simulink model "EdgeDetect"  (R2018b)
settings: Solver=VariableStepAuto  StartTime=0.0  StopTime=(64*3)*320e-9  RelTol=1e-3
libraries: xbsIndex_r4 x16, simulink_extras x2
settings Model: Creator=marsiau  LastModifiedBy=marsiau

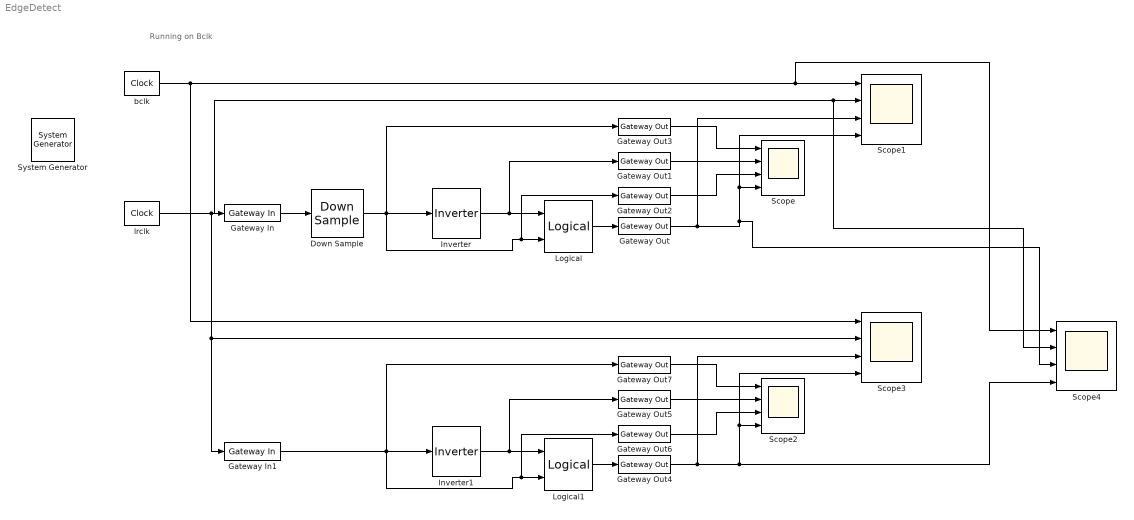
== system EdgeDetect ==
  note: Running on Bclk
  " System Generator" : xbsIndex_r4/ System Generator  Tag=genX  xilinxfamily=zynq  part=xc7z020  speed=-1  package=clg400  synthesis_tool=Vivado  clock_wrapper=Clock Enables  directory=./netlist  proj_type=Vivado  Synth_file=Vivado Synthesis Defaults  Impl_file=Vivado Implementation Defaults  testbench=off  simulink_period=320e-9  sysclk_period=320  dcm_input_clock_period=10  incr_netlist=off  trim_vbits=Everywhere in SubSystem  dbl_ovrd=According to Block Masks  core_generation=According to Block Masks  run_coregen=off  deprecated_control=off  eval_field=0  block_type=sysgen
  Down Sample : xbsIndex_r4/Down Sample  sample_ratio=32  sample_phase="Last Value of Frame  (most efficient)"  en=off  rst=off  latency=1  dbl_ovrd=off  block_type=dsamp
  Gateway In : xbsIndex_r4/Gateway In  gui_display_data_type=Boolean  arith_type=Boolean  n_bits=16  bin_pt=14  preci_type=Single  exp_width=8  frac_width=24  rows=1  columns=1  quantization="Round  (unbiased: +/- Inf)"  overflow=Saturate  period=320e-9  UseAsADC=off  ADCChannel='1'  interface=None  automatic_assignment=on  address_offset=hex2dec('00')  intf_name=''  intf_description=''  default_value=0  timing_constraint=None  locs_specified=off  LOCs={}  io_standard={}  inherit_from_input=off  hdl_port=on  dbl_ovrd=off  block_type=gatewayin
  Gateway In1 : xbsIndex_r4/Gateway In  gui_display_data_type=Boolean  arith_type=Boolean  n_bits=16  bin_pt=14  preci_type=Single  exp_width=8  frac_width=24  rows=1  columns=1  quantization="Round  (unbiased: +/- Inf)"  overflow=Saturate  period=320e-9  UseAsADC=off  ADCChannel='1'  interface=None  automatic_assignment=on  address_offset=hex2dec('00')  intf_name=''  intf_description=''  default_value=0  timing_constraint=None  locs_specified=off  LOCs={}  io_standard={}  inherit_from_input=off  hdl_port=on  dbl_ovrd=off  block_type=gatewayin
  Gateway Out{,1..7} (8 alike) : xbsIndex_r4/Gateway Out  inherit_from_input=off  hdl_port=on  rows=1  columns=1  UseAsDAC=off  DACChannel='1'  interface=None  automatic_assignment=on  address_offset=hex2dec('00')  intf_name=''  intf_description=''  timing_constraint=None  locs_specified=off  LOCs={}  io_standard={}  block_type=gatewayout
  Inverter : xbsIndex_r4/Inverter  en=off  latency=1  dbl_ovrd=off  block_type=inv
  Inverter1 : xbsIndex_r4/Inverter  en=off  latency=1  dbl_ovrd=off  block_type=inv
  Logical : xbsIndex_r4/Logical  logical_function=AND  inputs=2  en=off  latency=1  precision=Full  arith_type=Unsigned  n_bits=16  bin_pt=0  align_bp=on  dbl_ovrd=off  block_type=logical
  Logical1 : xbsIndex_r4/Logical  logical_function=AND  inputs=2  en=off  latency=1  precision=Full  arith_type=Unsigned  n_bits=16  bin_pt=0  align_bp=on  dbl_ovrd=off  block_type=logical
  Scope{,1..4} (5 alike) : Scope  NumInputPorts=4
  bclk : simulink_extras/Flip Flops/Clock  period=320e-9
  lrclk : simulink_extras/Flip Flops/Clock  period=20.48e-6
  wires:
  Logical/1 -> Gateway Out/1
  Inverter/1 -> Gateway Out1/1, Logical/1
  Gateway In/1 -> Down Sample/1
  Gateway Out3/1 -> Scope/1
  Gateway Out1/1 -> Scope/2
  Gateway Out2/1 -> Scope/3
  Down Sample/1 -> Gateway Out2/1, Logical/2, Inverter/1, Gateway Out3/1
  Inverter1/1 -> Gateway Out5/1, Logical1/1
  lrclk/1 -> Scope3/2, Gateway In1/1, Scope4/2, Scope1/2, Gateway In/1
  Gateway Out6/1 -> Scope2/3
  Logical1/1 -> Gateway Out4/1
  Gateway Out4/1 -> Scope3/3, Scope4/4, Scope3/4, Scope2/4
  Gateway Out7/1 -> Scope2/1
  Gateway Out5/1 -> Scope2/2
  Gateway In1/1 -> Gateway Out6/1, Logical1/2, Inverter1/1, Gateway Out7/1
  bclk/1 -> Scope3/1, Scope4/1, Scope1/1
  Gateway Out/1 -> Scope1/3, Scope4/3, Scope1/4, Scope/4
